simulink model "vsg1"  (R2014a)
settings: Solver=ode23tb  StartTime=0.0  StopTime=0.1  RelTol=1e-3
undefined symbols (not defined in the file): Ts
libraries: powerlib x6, powerlib_meascontrol x4
settings Model: Creator=ztg  LastModifiedBy=ztg

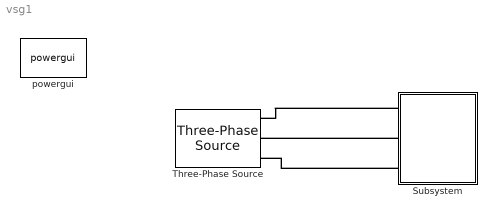
== system vsg1 ==
  Subsystem : Subsystem  mask{K=100, J=1, D=10}
      mask TypeOptions K: K/Gain
      mask TypeOptions J: J/Gain
      mask TypeOptions D: Dp/Gain
  Three-Phase Source : powerlib/Electrical Sources/Three-Phase Source  Voltage=1000*sqrt(2)  PhaseAngle=0  Frequency=50  InternalConnection=Yg  SpecifyImpedance=on  Resistance=0.8929  Inductance=16.58e-3  ShortCircuitLevel=100e6  BaseVoltage=25e3  XRratio=7  BusType=swing  Pref=0  Qref=0  Qmin=-inf  Qmax=inf
  powergui : powerlib/powergui  Priority=1  SimulationMode=Discrete  SolverType=Tustin  SampleTime=5e-5  frequency=60  SPID=off  DisableSnubberDevices=off  DisableRonSwitches=off  DisableVfSwitches=off  SwTol=0  Interpol=off  DisplayEquations=off  Ts=0  methode=off  frequencyindice=50  Pbase=100e6  ErrMax=1e-4  Iterations=50  UnitsV=kV  UnitsW=MW  FunctionMessages=off  echomessages=off  HookPort=off  EnableUseOfTLC=off  x0status=blocks  RestoreLinks=warning  ResistiveCurrentMeasurement=off  Frange=[0:2:500]  Ylog=off  Xlog=on  ShowGrid=off  save=off  variable=ZData  structure=0  ZoomFFT=off  StartTime=0.0  cycles=1  DisplayStyle=1  fundamental=60  FreqAxis=off  MaxFrequency=1000  frequencyindicesteady=1  RmsSteady=1  display=off
  connections:
  Subsystem/LConn1 -- Three-Phase Source/RConn1
  Subsystem/LConn2 -- Three-Phase Source/RConn2
  Subsystem/LConn3 -- Three-Phase Source/RConn3

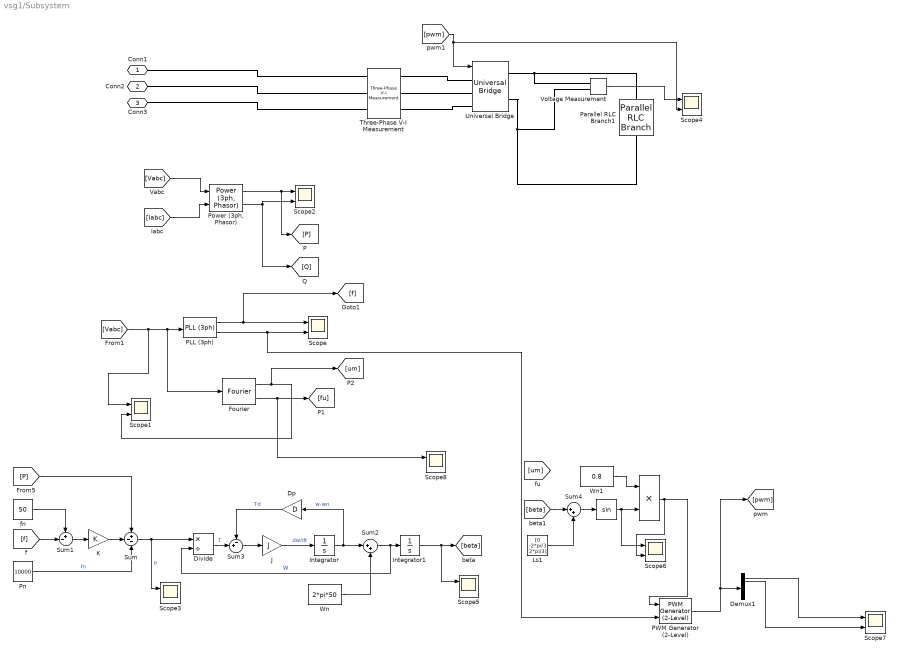
== system vsg1/Subsystem ==
  " " : Trigonometry
  "  " : Product
  Demux1 : Demux  Outputs=6
  Divide : Product  Inputs=*/
  Dp : Gain  Gain=D
  Fourier : powerlib_meascontrol/Measurements/Fourier  Freq=60  n=1  InInit=[0, 0]  Ts=Ts
  Integrator : Integrator
  Integrator1 : Integrator
  J : Gain  Gain=J
  K : Gain  Gain=K
  Ls1 : Constant  Value=[0 -2*pi/3 2*pi/3]
  PLL (3ph) : powerlib_meascontrol/PLL/PLL (3ph)  Fmin=45  Par_Init=[0, 60]  ParK=[180, 3200, 1]  TcD=1e-4  MaxRateChangeFreq=12  FilterCutOffFreq=25  Ts=0  AGC=on
  PWM Generator (2-Level) : powerlib_meascontrol/Pulse & Signal Generators/PWM Generator (2-Level)  ModulatorType=Three-phase bridge (6 pulses)  ModulatorMode=Synchronized  nF=27  Fc=27*50  ModulatingSignals=off  m=0.8  Freq=60  Phase=0  Ts=0
  Parallel RLC Branch1 : powerlib/Elements/Parallel RLC Branch  LConnTagsString=a  RConnTagsString=__new0  BranchType=R  Resistance=100  Inductance=1e-3  SetiL0=off  InitialCurrent=0  Capacitance=1e-6  Setx0=off  InitialVoltage=0  Measurements=None
  Pn : Constant  Value=10000
  "Power (3ph, Phasor)" : powerlib_meascontrol/Measurements/Power (3ph, Phasor)
  Scope{,1..8} (9 alike) : Scope  NumInputPorts=2
      Scope settings: YMin=59.9999~0  YMax=60~6.5
      Scope1 settings: YMin=-1200~0  YMax=1200~65
      Scope2 settings: YMin=0~-1  YMax=70000~1  SaveName=ScopeData2
      Scope3 settings: YMin=450~-1  YMax=1550~1  SaveName=ScopeData3
      Scope4 settings: YMin=-250~0  YMax=4000~1  SaveName=ScopeData4
      Scope5 settings: YMin=94~-1  YMax=113~1  SaveName=ScopeData5
      Scope6 settings: YMin=-1~-0.8  YMax=1~0.8  SaveName=ScopeData6
      Scope7 settings: TimeRange=0.001051620249093166  YMin=-0.5~-1  YMax=1.5~1  SaveName=ScopeData7
      Scope8 settings: YMin=-200~-1  YMax=200~1  SaveName=ScopeData8
  Sum : Sum  Inputs=+--
  Sum1 : Sum  Inputs=+-|
  Sum2 : Sum  Inputs=|++
  Sum3 : Sum  Inputs=-+|
  Sum4 : Sum  Inputs=|++
  Three-Phase V-I Measurement : powerlib/Measurements/Three-Phase V-I Measurement  VoltageMeasurement=phase-to-ground  SetLabelV=on  LabelV=Vabc  Vpu=off  VpuLL=off  CurrentMeasurement=yes  SetLabelI=on  LabelI=Iabc  Ipu=off  Pbase=100e6  Vbase=500e3  OutputType=Complex  PhasorSimulation=off  PSBequivalent=0
  Universal Bridge : powerlib/Power Electronics/Universal Bridge  Arms=3  SnubberResistance=1e5  SnubberCapacitance=inf  Device=IGBT / Diodes  Ron=1e-3  Lon=0  ForwardVoltages="[  0  0  ]"  ForwardVoltage=0  GTOparameters=[ 10e-6 , 20e-6 ]  IGBTparameters=[ 1e-6 , 2e-6 ]  Measurements=None  Measurements_2=None  converterType=Rectifier
  Voltage Measurement : powerlib/Measurements/Voltage Measurement  PhasorSimulation=off  OutputType=Complex  PSBequivalent=0
  Wn : Constant  Value=2*pi*50
  Wn1 : Constant  Value=0.8
  fn : Constant  Value=50
  Conn1 : PMIOPort  Port=1  Side=Left
  Conn2 : PMIOPort  Port=2  Side=Left
  Conn3 : PMIOPort  Port=3  Side=Left
  wires:
  [Vabc] -> Fourier/1, PLL (3ph)/1, Scope1/1
  PLL (3ph)/1 -> [f], Scope/1
  PLL (3ph)/2 -> PWM Generator (2-Level)/2, Scope/2
  Fourier/1 -> [um], Scope1/2
  [Vabc] -> "Power (3ph, Phasor)"/1
  [Iabc] -> "Power (3ph, Phasor)"/2
  "Power (3ph, Phasor)"/1 -> [P], Scope2/1
  "Power (3ph, Phasor)"/2 -> [Q], Scope2/2
  Voltage Measurement/1 -> Scope4/1
  [P] -> Sum/1
  [f] -> Sum1/2
  fn/1 -> Sum1/1
  K/1 -> Sum/2
  Sum1/1 -> K/1
  Pn/1 -> Sum/3  "fn"
  Sum/1 -> Divide/1, Scope3/1  "P"
  J/1 -> Integrator/1  "dw/dt"
  Wn/1 -> Sum2/2
  Dp/1 -> Sum3/1  "Td"
  Divide/1 -> Sum3/2  "T"
  Sum3/1 -> J/1
  Sum2/1 -> Divide/2, Integrator1/1  "W"
  Integrator1/1 -> Scope5/1, [beta]
  [pwm] -> Scope4/2, Universal Bridge/1
  Fourier/2 -> Scope8/1, [fu]
  Sum4/1 -> " "/1
  [beta] -> Sum4/1
  Ls1/1 -> Sum4/2
  " "/1 -> Scope6/1, "  "/2
  Integrator/1 -> Sum2/1, Dp/1  "w-wn"
  "  "/1 -> Scope6/2, PWM Generator (2-Level)/1
  Wn1/1 -> "  "/1
  PWM Generator (2-Level)/1 -> [pwm], Demux1/1
  ? -> ?
  Demux1/1 -> Scope7/1
  Demux1/2 -> Scope7/2
  connections:
  Universal Bridge/RConn1 -- Voltage Measurement/LConn1 -- Parallel RLC Branch1/LConn1
  Universal Bridge/RConn2 -- Voltage Measurement/LConn2 -- Parallel RLC Branch1/RConn1
  Conn1/RConn1 -- Three-Phase V-I Measurement/LConn1
  Conn2/RConn1 -- Three-Phase V-I Measurement/LConn2
  Conn3/RConn1 -- Three-Phase V-I Measurement/LConn3
  Three-Phase V-I Measurement/RConn2 -- Universal Bridge/LConn2
  Three-Phase V-I Measurement/RConn1 -- Universal Bridge/LConn1
  Three-Phase V-I Measurement/RConn3 -- Universal Bridge/LConn3
